simulink subsystem "Gearbox"  (R2023a)
settings: Solver=VariableStepAuto  StartTime=0.0  StopTime=10.0  RelTol=1e-3
values from neighbouring files (symbols this model uses):
  a = 0.001    [main.m]
  c = 2000000    [main.m]
  F1 = 0    [main.m]
  F2 = 0    [main.m]
  G = 0    [main.m]
  G1 = 0    [main.m]
  G2 = 0    [main.m]
  i = 100    [main.m]
  J = 0.04    [main.m]
settings Model: Creator=ycheb  LastModifiedBy=ycheb

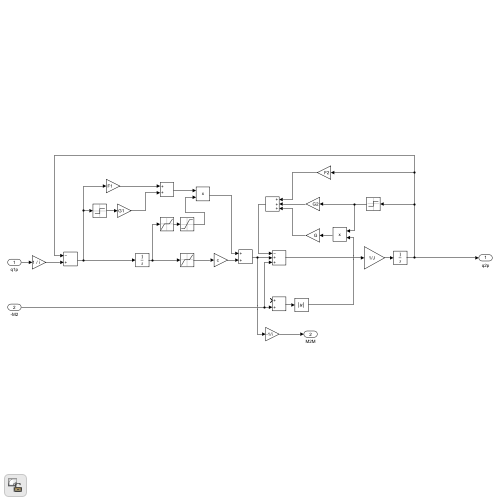
[thumbnail: Simulink's stored preview of the top-level diagram]
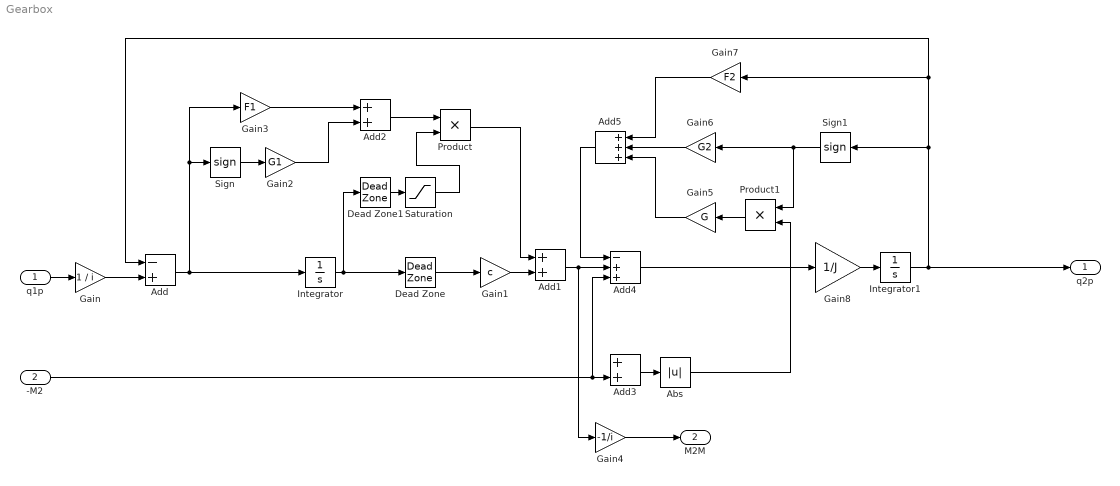
== system Gearbox ==
  q1p : Inport
  -M2 : Inport  Port=2
  Abs : Abs  SaturateOnIntegerOverflow=off
  Add : Sum  Inputs=-+
  Add1 : Sum
  Add2 : Sum
  Add3 : Sum
  Add4 : Sum  Inputs=-++
  Add5 : Sum  Inputs=+++
  Dead Zone : DeadZone  LowerValue=-a  UpperValue=a
  Dead Zone1 : DeadZone  LowerValue=-a  UpperValue=a
  Gain : Gain  Gain=1 / i
  Gain1 : Gain  Gain=c
  Gain2 : Gain  Gain=G1
  Gain3 : Gain  Gain=F1
  Gain4 : Gain  Gain=-1/i
  Gain5 : Gain  Gain=G
  Gain6 : Gain  Gain=G2
  Gain7 : Gain  Gain=F2
  Gain8 : Gain  Gain=1/J
  Integrator : Integrator
  Integrator1 : Integrator
  Product : Product
  Product1 : Product
  Saturation : Saturate  UpperLimit=a  LowerLimit=-a
  Sign : Signum
  Sign1 : Signum
  q2p : Outport
  M2M : Outport  Port=2
  wires:
  q1p/1 -> Gain/1
  Gain/1 -> Add/2
  Add/1 -> Integrator/1, Sign/1, Gain3/1
  Integrator/1 -> Dead Zone/1, Dead Zone1/1
  Dead Zone/1 -> Gain1/1
  Gain1/1 -> Add1/2
  Dead Zone1/1 -> Saturation/1
  Saturation/1 -> Product/2
  Product/1 -> Add1/1
  Add2/1 -> Product/1
  Gain2/1 -> Add2/2
  Sign/1 -> Gain2/1
  Gain3/1 -> Add2/1
  -M2/1 -> Add3/2, Add4/3
  Add1/1 -> Add4/2, Gain4/1
  Gain4/1 -> M2M/1
  Add3/1 -> Abs/1
  Add5/1 -> Add4/1
  Product1/1 -> Gain5/1
  Gain5/1 -> Add5/3
  Abs/1 -> Product1/2
  Gain6/1 -> Add5/2
  Sign1/1 -> Gain6/1, Product1/1
  Gain7/1 -> Add5/1
  Add4/1 -> Gain8/1
  Gain8/1 -> Integrator1/1
  Integrator1/1 -> q2p/1, Sign1/1, Gain7/1, Add/1
